simulink model "dynamic_for_landing1"  (Simulink 8.0)
settings: Solver=ode4  StartTime=0.0  StopTime=500  FixedStep=0.1  RelTol=1e-3
values from neighbouring files (symbols this model uses):
  AA = [Wex^2-W^2   Wex*Wey    Wex*Wez ... (first row only)    [main4_cvx_land.m]    (also in ss.mat = [0  0  0; 0  -1.096815312e-07  0; 0  0  -1.096815312e-07])
  BB = [   0    -2*Wez    2*Wey ... (first row only)    [main4_cvx_land.m]    (also in ss.mat = [0  0  0; 0  0  0.000662364042503; 0  -0.000662364042503  0])
  c20 = -0.113    [get_U.m]    (also in main4_cvx_land.m; ss.mat)
  c22 = 0.0396    [get_U.m]    (also in main4_cvx_land.m; ss.mat)
  Gl = [cos(xit0)*sin(fai0)   sin(xit0)*sin(fai0)    -cos(fai0) ... (first row only)    [main4_cvx_land.m]    (also in ss.mat = [0  -0.995743716786  0.0921653431654; 0  0.0921653431654  0.)
  Mu = 4.794e3    (= 4794)    [get_U.m]    (also in main4_cvx_land.m; ss.mat)
  r0 = RV_result(1:3)    [main4_cvx_land.m]    (also in ss.mat = [0.00818770646738 -0.0171318118409 0.193514552177])
  re = 1750    [get_U.m]    (also in main4_cvx_land.m; ss.mat)
  rol = [0;0;R0l]    [main4_cvx_land.m]    (also in ss.mat = [0 0 5423.1])
  uu = XX(6*(p+1)+1:6*(p+1)+3)    [main4_cvx_land.m]    (also in ss.mat = [5.11203407339e-05 2.7599566741e-06 -0.000430545373227])
  v0 = RV_result(4:6)    [main4_cvx_land.m]    (also in ss.mat = [-0.00102833647286 0.000389600939224 0.00135850795722])
undefined symbols (not defined in the file or in its folder): magnitude
settings Model: Creator=Administrator  LastModifiedBy=Administrator
settings OptimizationCC: ExpressionDepthLimit=128
settings DebuggingCC: UnderspecifiedInitializationDetection=Simplified  StateNameClashWarn=none
settings CodeAppCC: CustomSymbolStrType=$N$R$M_T  InternalIdentifier=Shortened
settings GRTTargetCC: CodeReplacementLibrary=None  CPPClassGenCompliant=on

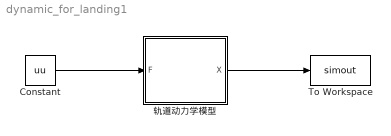
== system dynamic_for_landing1 ==
  Constant : Constant  Value=uu
  To Workspace : ToWorkspace  VariableName=simout  SampleTime=-1
  轨道动力学模型 : Subsystem
      mask help:
      | 输入:
      | 喷嘴产生的推力(特征点坐标系)
      | 输出:
      | 1、探测器的位置与速度(特征点坐标系)
      | 2、比力(特征点坐标系)
      mask Display: disp('轨道动力学模型')
  wires:
  Constant/1 -> 轨道动力学模型/1(F)
  轨道动力学模型/1(X) -> To Workspace/1

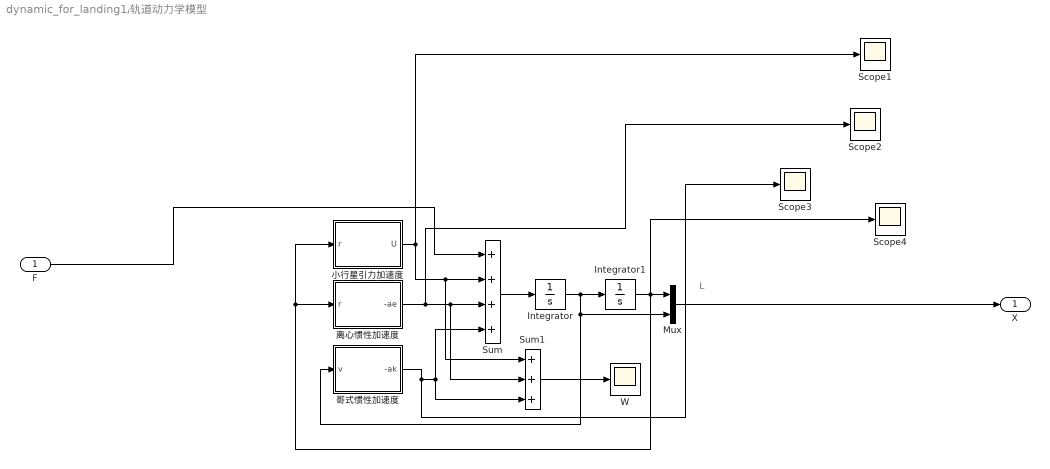
== system dynamic_for_landing1/轨道动力学模型 ==
  note: L
  F : Inport
  Integrator : Integrator  InitialCondition=v0
  Integrator1 : Integrator  InitialCondition=r0
  Mux : Mux  Inputs=2
  Scope{1..4} (4 alike) : Scope
  Sum : Sum  Inputs=++++  SaturateOnIntegerOverflow=on
  Sum1 : Sum  Inputs=+++  SaturateOnIntegerOverflow=on
  W : Scope
  哥式惯性加速度 : Subsystem
  小行星引力加速度 : Subsystem
  离心惯性加速度 : Subsystem
  X : Outport
  wires:
  Sum1/1 -> W/1
  Integrator1/1 -> 小行星引力加速度/1(r), 离心惯性加速度/1(r), Mux/1, Scope4/1
  Mux/1 -> X/1
  Integrator/1 -> 哥式惯性加速度/1(v), Mux/2, Integrator1/1
  Sum/1 -> Integrator/1
  哥式惯性加速度/1(-ak) -> Sum1/3, Sum/4, Scope3/1
  离心惯性加速度/1(-ae) -> Sum1/2, Sum/3, Scope2/1
  小行星引力加速度/1(U) -> Scope1/1, Sum1/1, Sum/2
  F/1 -> Sum/1

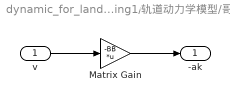
== system dynamic_for_landing1/轨道动力学模型/哥式惯性加速度 ==
  v : Inport
  Matrix Gain : Gain  Gain=-BB  Multiplication=Matrix(K*u)  SaturateOnIntegerOverflow=on  OutDataTypeStr=Inherit: Same as input  ParamDataTypeStr=Inherit: Same as input
  -ak : Outport
  wires:
  Matrix Gain/1 -> -ak/1
  v/1 -> Matrix Gain/1

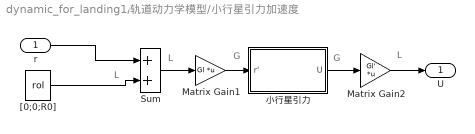
== system dynamic_for_landing1/轨道动力学模型/小行星引力加速度 ==
  note: L
  note: L
  note: G
  note: G
  note: L
  r : Inport
  Matrix Gain1 : Gain  Gain=Gl  Multiplication=Matrix(K*u)  SaturateOnIntegerOverflow=on  OutDataTypeStr=Inherit: Same as input  ParamDataTypeStr=Inherit: Same as input
  Matrix Gain2 : Gain  Gain=Gl'  Multiplication=Matrix(K*u)  SaturateOnIntegerOverflow=on  OutDataTypeStr=Inherit: Same as input  ParamDataTypeStr=Inherit: Same as input
  Sum : Sum  SaturateOnIntegerOverflow=on
  "[0;0;R0]" : Constant  Value=rol
  小行星引力 : Subsystem
      mask Display: disp('小行星引力')
  U : Outport
  wires:
  Matrix Gain2/1 -> U/1
  小行星引力/1(U) -> Matrix Gain2/1
  Matrix Gain1/1 -> 小行星引力/1(r')
  Sum/1 -> Matrix Gain1/1
  r/1 -> Sum/1
  "[0;0;R0]"/1 -> Sum/2

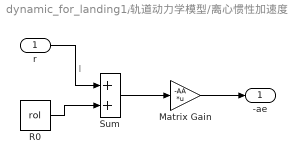
== system dynamic_for_landing1/轨道动力学模型/离心惯性加速度 ==
  note: l
  r : Inport
  Matrix Gain : Gain  Gain=-AA  Multiplication=Matrix(K*u)  SaturateOnIntegerOverflow=on  OutDataTypeStr=Inherit: Same as input  ParamDataTypeStr=Inherit: Same as input
  R0 : Constant  Value=rol
  Sum : Sum  SaturateOnIntegerOverflow=on
  -ae : Outport
  wires:
  Matrix Gain/1 -> -ae/1
  Sum/1 -> Matrix Gain/1
  r/1 -> Sum/1
  R0/1 -> Sum/2

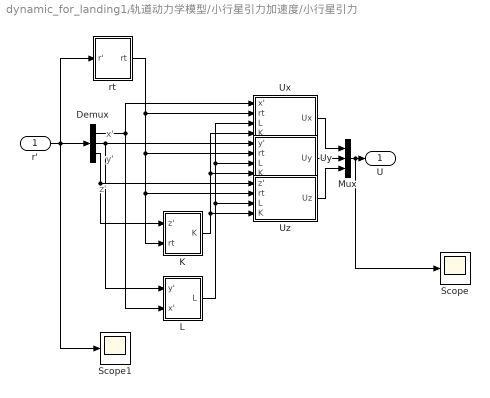
== system dynamic_for_landing1/轨道动力学模型/小行星引力加速度/小行星引力 ==
  note: x'
  note: y'
  note: z'
  r' : Inport
  Demux : Demux  Outputs=3
  K : Subsystem
  L : Subsystem
  Mux : Mux  Inputs=3
  Scope : Scope
  Scope1 : Scope
  Ux : Subsystem
  Uy : Subsystem
  Uz : Subsystem
  rt : Subsystem
  U : Outport
  wires:
  L/1(L) -> Uy/3(L), Ux/3(L), Uz/3(L)
  K/1(K) -> Uy/4(K), Ux/4(K), Uz/4(K)
  Demux/2 -> L/1(y'), Uy/1(y')
  Demux/3 -> K/1(z'), Uz/1(z')
  rt/1(rt) -> Uy/2(rt), K/2(rt), Uz/2(rt), Ux/2(rt)
  Uz/1(Uz) -> Mux/3
  Ux/1(Ux) -> Mux/1
  Uy/1(Uy) -> Mux/2
  Mux/1 -> U/1, Scope/1
  r'/1 -> rt/1(r'), Demux/1, Scope1/1
  Demux/1 -> L/2(x'), Ux/1(x')

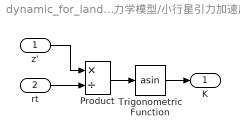
== system dynamic_for_landing1/轨道动力学模型/小行星引力加速度/小行星引力/K ==
  z' : Inport
  rt : Inport  Port=2
  Product : Product  Inputs=*/  SaturateOnIntegerOverflow=on  OutDataTypeStr=Inherit: Same as first input
  Trigonometric Function : Trigonometry  Operator=asin
  K : Outport
  wires:
  Product/1 -> Trigonometric Function/1
  rt/1 -> Product/2
  z'/1 -> Product/1
  Trigonometric Function/1 -> K/1

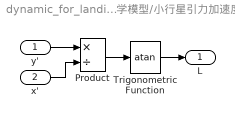
== system dynamic_for_landing1/轨道动力学模型/小行星引力加速度/小行星引力/L ==
  y' : Inport
  x' : Inport  Port=2
  Product : Product  Inputs=*/  SaturateOnIntegerOverflow=on  OutDataTypeStr=Inherit: Same as first input
  Trigonometric Function : Trigonometry  Operator=atan
  L : Outport
  wires:
  Trigonometric Function/1 -> L/1
  x'/1 -> Product/2
  y'/1 -> Product/1
  Product/1 -> Trigonometric Function/1

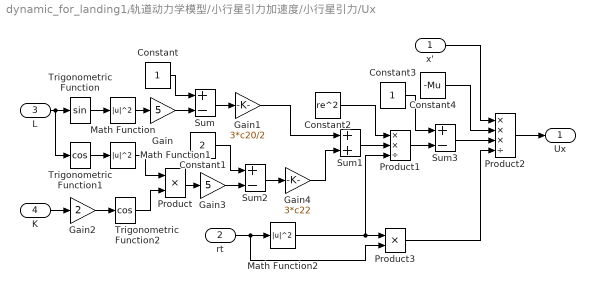
== system dynamic_for_landing1/轨道动力学模型/小行星引力加速度/小行星引力/Ux ==
  x' : Inport
  rt : Inport  Port=2
  L : Inport  Port=3
  K : Inport  Port=4
  Constant : Constant
  Constant1 : Constant  Value=2
  Constant2 : Constant  Value=re^2
  Constant3 : Constant
  Constant4 : Constant  Value=-Mu
  Gain : Gain  Gain=5  SaturateOnIntegerOverflow=on  OutDataTypeStr=Inherit: Same as input  ParamDataTypeStr=Inherit: Same as input
  Gain1 : Gain  Gain=3*c20/2  SaturateOnIntegerOverflow=on  OutDataTypeStr=Inherit: Same as input  ParamDataTypeStr=Inherit: Same as input
  Gain2 : Gain  Gain=2  SaturateOnIntegerOverflow=on  OutDataTypeStr=Inherit: Same as input  ParamDataTypeStr=Inherit: Same as input
  Gain3 : Gain  Gain=5  SaturateOnIntegerOverflow=on  OutDataTypeStr=Inherit: Same as input  ParamDataTypeStr=Inherit: Same as input
  Gain4 : Gain  Gain=3*c22  SaturateOnIntegerOverflow=on  OutDataTypeStr=Inherit: Same as input  ParamDataTypeStr=Inherit: Same as input
  Math Function : Math  Operator=magnitude^2  SaturateOnIntegerOverflow=on
  Math Function1 : Math  Operator=magnitude^2  SaturateOnIntegerOverflow=on
  Math Function2 : Math  Operator=magnitude^2  SaturateOnIntegerOverflow=on
  Product : Product  SaturateOnIntegerOverflow=on  OutDataTypeStr=Inherit: Same as first input
  Product1 : Product  Inputs=**/  SaturateOnIntegerOverflow=on  OutDataTypeStr=Inherit: Same as first input
  Product2 : Product  Inputs=***/  SaturateOnIntegerOverflow=on  OutDataTypeStr=Inherit: Same as first input
  Product3 : Product  SaturateOnIntegerOverflow=on  OutDataTypeStr=Inherit: Same as first input
  Sum : Sum  Inputs=+-  SaturateOnIntegerOverflow=on
  Sum1 : Sum  SaturateOnIntegerOverflow=on
  Sum2 : Sum  Inputs=+-  SaturateOnIntegerOverflow=on
  Sum3 : Sum  Inputs=+-  SaturateOnIntegerOverflow=on
  Trigonometric Function : Trigonometry
  Trigonometric Function1 : Trigonometry  Operator=cos
  Trigonometric Function2 : Trigonometry  Operator=cos
  Ux : Outport
  wires:
  Product2/1 -> Ux/1
  Product3/1 -> Product2/4
  x'/1 -> Product2/1
  Constant4/1 -> Product2/2
  Sum3/1 -> Product2/3
  Constant3/1 -> Sum3/1
  Product1/1 -> Sum3/2
  Constant2/1 -> Product1/1
  Math Function2/1 -> Product3/1, Product1/3
  Sum1/1 -> Product1/2
  rt/1 -> Product3/2, Math Function2/1
  Gain1/1 -> Sum1/1
  Gain4/1 -> Sum1/2
  Sum2/1 -> Gain4/1
  Gain3/1 -> Sum2/2
  Constant1/1 -> Sum2/1
  Product/1 -> Gain3/1
  Math Function1/1 -> Product/1
  Trigonometric Function2/1 -> Product/2
  Gain2/1 -> Trigonometric Function2/1
  K/1 -> Gain2/1
  Trigonometric Function1/1 -> Math Function1/1
  Sum/1 -> Gain1/1
  Gain/1 -> Sum/2
  Constant/1 -> Sum/1
  Math Function/1 -> Gain/1
  Trigonometric Function/1 -> Math Function/1
  L/1 -> Trigonometric Function1/1, Trigonometric Function/1

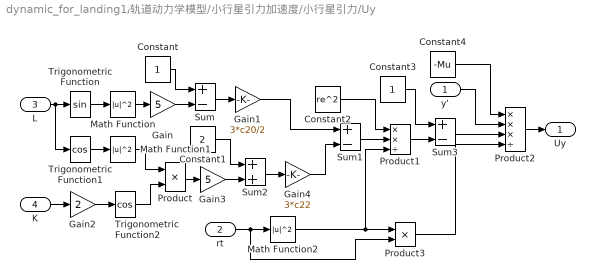
== system dynamic_for_landing1/轨道动力学模型/小行星引力加速度/小行星引力/Uy ==
  y' : Inport
  rt : Inport  Port=2
  L : Inport  Port=3
  K : Inport  Port=4
  Constant : Constant
  Constant1 : Constant  Value=2
  Constant2 : Constant  Value=re^2
  Constant3 : Constant
  Constant4 : Constant  Value=-Mu
  Gain : Gain  Gain=5  SaturateOnIntegerOverflow=on  OutDataTypeStr=Inherit: Same as input  ParamDataTypeStr=Inherit: Same as input
  Gain1 : Gain  Gain=3*c20/2  SaturateOnIntegerOverflow=on  OutDataTypeStr=Inherit: Same as input  ParamDataTypeStr=Inherit: Same as input
  Gain2 : Gain  Gain=2  SaturateOnIntegerOverflow=on  OutDataTypeStr=Inherit: Same as input  ParamDataTypeStr=Inherit: Same as input
  Gain3 : Gain  Gain=5  SaturateOnIntegerOverflow=on  OutDataTypeStr=Inherit: Same as input  ParamDataTypeStr=Inherit: Same as input
  Gain4 : Gain  Gain=3*c22  SaturateOnIntegerOverflow=on  OutDataTypeStr=Inherit: Same as input  ParamDataTypeStr=Inherit: Same as input
  Math Function : Math  Operator=magnitude^2  SaturateOnIntegerOverflow=on
  Math Function1 : Math  Operator=magnitude^2  SaturateOnIntegerOverflow=on
  Math Function2 : Math  Operator=magnitude^2  SaturateOnIntegerOverflow=on
  Product : Product  SaturateOnIntegerOverflow=on  OutDataTypeStr=Inherit: Same as first input
  Product1 : Product  Inputs=**/  SaturateOnIntegerOverflow=on  OutDataTypeStr=Inherit: Same as first input
  Product2 : Product  Inputs=***/  SaturateOnIntegerOverflow=on  OutDataTypeStr=Inherit: Same as first input
  Product3 : Product  SaturateOnIntegerOverflow=on  OutDataTypeStr=Inherit: Same as first input
  Sum : Sum  Inputs=+-  SaturateOnIntegerOverflow=on
  Sum1 : Sum  Inputs=+-  SaturateOnIntegerOverflow=on
  Sum2 : Sum  SaturateOnIntegerOverflow=on
  Sum3 : Sum  Inputs=+-  SaturateOnIntegerOverflow=on
  Trigonometric Function : Trigonometry
  Trigonometric Function1 : Trigonometry  Operator=cos
  Trigonometric Function2 : Trigonometry  Operator=cos
  Uy : Outport
  wires:
  Product3/1 -> Product2/4
  Sum3/1 -> Product2/3
  Constant4/1 -> Product2/1
  y'/1 -> Product2/2
  Product2/1 -> Uy/1
  Constant3/1 -> Sum3/1
  Product1/1 -> Sum3/2
  Constant2/1 -> Product1/1
  Math Function2/1 -> Product3/1, Product1/3
  Sum1/1 -> Product1/2
  rt/1 -> Product3/2, Math Function2/1
  Gain1/1 -> Sum1/1
  Gain4/1 -> Sum1/2
  Sum2/1 -> Gain4/1
  Gain3/1 -> Sum2/2
  Constant1/1 -> Sum2/1
  Product/1 -> Gain3/1
  Math Function1/1 -> Product/1
  Trigonometric Function2/1 -> Product/2
  Gain2/1 -> Trigonometric Function2/1
  K/1 -> Gain2/1
  Trigonometric Function1/1 -> Math Function1/1
  Sum/1 -> Gain1/1
  Gain/1 -> Sum/2
  Constant/1 -> Sum/1
  Math Function/1 -> Gain/1
  Trigonometric Function/1 -> Math Function/1
  L/1 -> Trigonometric Function1/1, Trigonometric Function/1

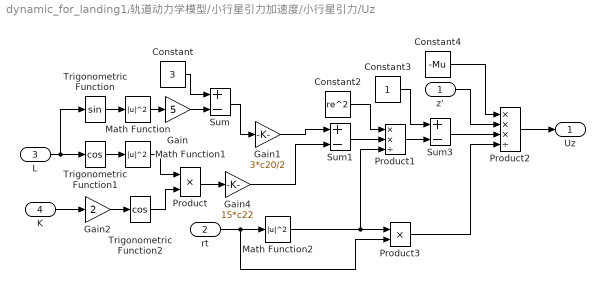
== system dynamic_for_landing1/轨道动力学模型/小行星引力加速度/小行星引力/Uz ==
  z' : Inport
  rt : Inport  Port=2
  L : Inport  Port=3
  K : Inport  Port=4
  Constant : Constant  Value=3
  Constant2 : Constant  Value=re^2
  Constant3 : Constant
  Constant4 : Constant  Value=-Mu
  Gain : Gain  Gain=5  SaturateOnIntegerOverflow=on  OutDataTypeStr=Inherit: Same as input  ParamDataTypeStr=Inherit: Same as input
  Gain1 : Gain  Gain=3*c20/2  SaturateOnIntegerOverflow=on  OutDataTypeStr=Inherit: Same as input  ParamDataTypeStr=Inherit: Same as input
  Gain2 : Gain  Gain=2  SaturateOnIntegerOverflow=on  OutDataTypeStr=Inherit: Same as input  ParamDataTypeStr=Inherit: Same as input
  Gain4 : Gain  Gain=15*c22  SaturateOnIntegerOverflow=on  OutDataTypeStr=Inherit: Same as input  ParamDataTypeStr=Inherit: Same as input
  Math Function : Math  Operator=magnitude^2  SaturateOnIntegerOverflow=on
  Math Function1 : Math  Operator=magnitude^2  SaturateOnIntegerOverflow=on
  Math Function2 : Math  Operator=magnitude^2  SaturateOnIntegerOverflow=on
  Product : Product  SaturateOnIntegerOverflow=on  OutDataTypeStr=Inherit: Same as first input
  Product1 : Product  Inputs=**/  SaturateOnIntegerOverflow=on  OutDataTypeStr=Inherit: Same as first input
  Product2 : Product  Inputs=***/  SaturateOnIntegerOverflow=on  OutDataTypeStr=Inherit: Same as first input
  Product3 : Product  SaturateOnIntegerOverflow=on  OutDataTypeStr=Inherit: Same as first input
  Sum : Sum  Inputs=+-  SaturateOnIntegerOverflow=on
  Sum1 : Sum  Inputs=+-  SaturateOnIntegerOverflow=on
  Sum3 : Sum  Inputs=+-  SaturateOnIntegerOverflow=on
  Trigonometric Function : Trigonometry
  Trigonometric Function1 : Trigonometry  Operator=cos
  Trigonometric Function2 : Trigonometry  Operator=cos
  Uz : Outport
  wires:
  Product2/1 -> Uz/1
  Gain4/1 -> Sum1/2
  L/1 -> Trigonometric Function/1, Trigonometric Function1/1
  K/1 -> Gain2/1
  Product3/1 -> Product2/4
  Sum3/1 -> Product2/3
  Constant4/1 -> Product2/1
  z'/1 -> Product2/2
  Constant3/1 -> Sum3/1
  Product1/1 -> Sum3/2
  Constant2/1 -> Product1/1
  Math Function2/1 -> Product3/1, Product1/3
  Sum1/1 -> Product1/2
  rt/1 -> Product3/2, Math Function2/1
  Gain1/1 -> Sum1/1
  Product/1 -> Gain4/1
  Math Function1/1 -> Product/1
  Trigonometric Function2/1 -> Product/2
  Gain2/1 -> Trigonometric Function2/1
  Trigonometric Function1/1 -> Math Function1/1
  Sum/1 -> Gain1/1
  Gain/1 -> Sum/2
  Constant/1 -> Sum/1
  Math Function/1 -> Gain/1
  Trigonometric Function/1 -> Math Function/1

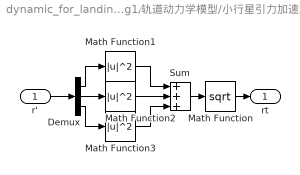
== system dynamic_for_landing1/轨道动力学模型/小行星引力加速度/小行星引力/rt ==
  r' : Inport
  Demux : Demux  Outputs=3
  Math Function : Math  Operator=sqrt  SaturateOnIntegerOverflow=on
  Math Function1 : Math  Operator=magnitude^2  SaturateOnIntegerOverflow=on
  Math Function2 : Math  Operator=magnitude^2  SaturateOnIntegerOverflow=on
  Math Function3 : Math  Operator=magnitude^2  SaturateOnIntegerOverflow=on
  Sum : Sum  Inputs=+++  SaturateOnIntegerOverflow=on
  rt : Outport
  wires:
  Math Function3/1 -> Sum/3
  Math Function2/1 -> Sum/2
  Math Function1/1 -> Sum/1
  Sum/1 -> Math Function/1
  Math Function/1 -> rt/1
  Demux/3 -> Math Function3/1
  Demux/2 -> Math Function2/1
  Demux/1 -> Math Function1/1
  r'/1 -> Demux/1
